simulink model "exp_dcMotor_simulink"  (R2016a)
settings: Solver=VariableStepAuto  SolverMode=SingleTasking  StartTime=0.0  StopTime=10.0  RelTol=1e-3
libraries: simulink x5
settings Model: Creator=Igor  LastModifiedBy=david
settings DebuggingCC: SFUnexpectedBacktrackingDiag=error  SFNoUnconditionalDefaultTransitionDiag=error
settings GRTTargetCC: TargetLangStandard=C99 (ISO)  GeneratePreprocessorConditionals=Use local settings
settings ConfigComp: CovMetricSettings=dwe  CovHtmlReporting=off  CovSaveCumulativeToWorkspaceVar=off  CovSaveSingleToWorkspaceVar=off  CovExternalEMLEnable=on

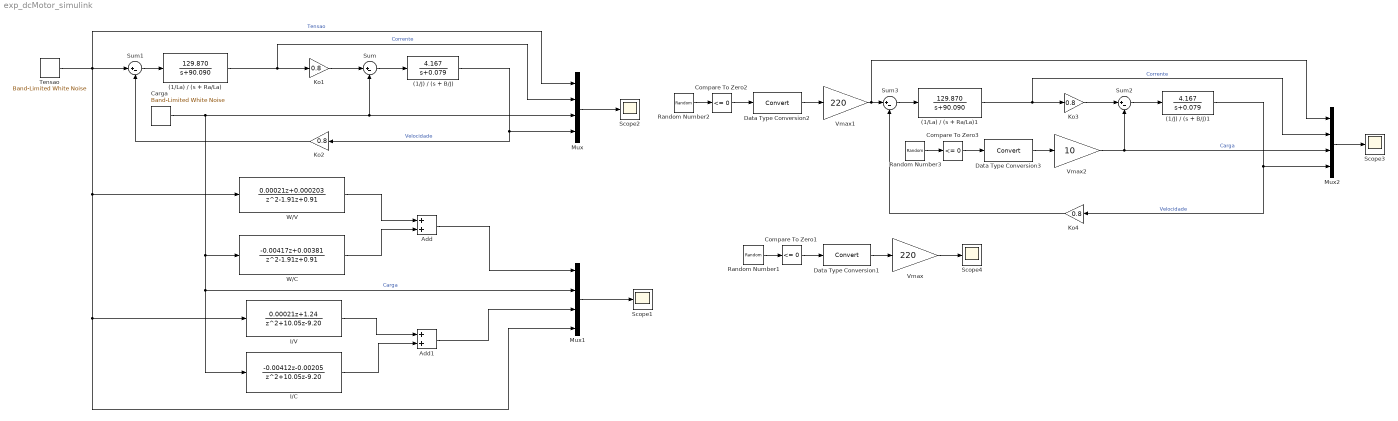
== system exp_dcMotor_simulink ==
  (1/J) / (s + B/J) : TransferFcn  Numerator=[4.167]  Denominator=[1 0.079]
  (1/J) / (s + B/J)1 : TransferFcn  Numerator=[4.167]  Denominator=[1 0.079]
  (1/La) / (s + Ra/La) : TransferFcn  Numerator=[129.870]  Denominator=[1 90.090 ]
  (1/La) / (s + Ra/La)1 : TransferFcn  Numerator=[129.870]  Denominator=[1 90.090 ]
  Add : Sum
  Add1 : Sum
  Carga : simulink/Sources/Band-Limited White Noise  Cov=[10]  Ts=0.001  seed=[23341]
  Compare To Zero1 : simulink/Logic and Bit Operations/Compare To Zero  relop=<=  OutDataTypeStr=uint8
  Compare To Zero2 : simulink/Logic and Bit Operations/Compare To Zero  relop=<=  OutDataTypeStr=uint8
  Compare To Zero3 : simulink/Logic and Bit Operations/Compare To Zero  relop=<=  OutDataTypeStr=uint8
  Data Type Conversion1 : DataTypeConversion
  Data Type Conversion2 : DataTypeConversion
  Data Type Conversion3 : DataTypeConversion
  I/C : DiscreteTransferFcn  Numerator=[-0.00412 -0.00205]  Denominator=[1 10.05 -9.20]
  "I/V " : DiscreteTransferFcn  Numerator=[0.00021 1.24]  Denominator=[1 10.05 -9.20]
  Ko{1..4} (4 alike) : Gain  Gain=0.8
  Mux : Mux
  Mux1 : Mux
  Mux2 : Mux
  Random Number1 : RandomNumber  SampleTime=0.001
  Random Number2 : RandomNumber  SampleTime=0.001
  Random Number3 : RandomNumber  SampleTime=0.001
  Scope{1..4} (4 alike) : Scope
  Sum{,1..3} (4 alike) : Sum  Inputs=|+-
  Tensao : simulink/Sources/Band-Limited White Noise  Cov=[100]  Ts=0.001  seed=[23342]
  Vmax : Gain  Gain=220
  Vmax1 : Gain  Gain=220
  Vmax2 : Gain  Gain=10
  "W/C " : DiscreteTransferFcn  Numerator=[-0.00417 0.00381]  Denominator=[1 -1.91 0.91]
  "W/V " : DiscreteTransferFcn  Numerator=[0.00021 0.000203]  Denominator=[1 -1.91 0.91]
  wires:
  Sum1/1 -> (1/La) / (s + Ra/La)/1
  (1/J) / (s + B/J)/1 -> Ko2/1, Mux/4  "Velocidade"
  Ko1/1 -> Sum/1
  Sum/1 -> (1/J) / (s + B/J)/1
  Ko2/1 -> Sum1/2
  Mux/1 -> Scope2/1
  "W/V "/1 -> Add/1
  "W/C "/1 -> Add/2
  Add/1 -> Mux1/1
  I/C/1 -> Add1/2
  "I/V "/1 -> Add1/1
  Mux1/1 -> Scope1/1
  Add1/1 -> Mux1/3
  Carga/1 -> I/C/1, Mux1/2, "W/C "/1, Sum/2, Mux/3  "Carga"
  Tensao/1 -> Mux/1, Sum1/1, "W/V "/1, Mux1/4, "I/V "/1  "Tensao"
  (1/La) / (s + Ra/La)/1 -> Ko1/1, Mux/2  "Corrente"
  Sum3/1 -> (1/La) / (s + Ra/La)1/1
  (1/J) / (s + B/J)1/1 -> Ko4/1, Mux2/4  "Velocidade"
  Ko3/1 -> Sum2/1
  Sum2/1 -> (1/J) / (s + B/J)1/1
  Ko4/1 -> Sum3/2
  Mux2/1 -> Scope3/1
  Vmax2/1 -> Sum2/2, Mux2/3  "Carga"
  (1/La) / (s + Ra/La)1/1 -> Ko3/1, Mux2/2  "Corrente"
  Random Number1/1 -> Compare To Zero1/1
  Vmax/1 -> Scope4/1
  Compare To Zero1/1 -> Data Type Conversion1/1
  Data Type Conversion1/1 -> Vmax/1
  Random Number2/1 -> Compare To Zero2/1
  Compare To Zero2/1 -> Data Type Conversion2/1
  Data Type Conversion2/1 -> Vmax1/1
  Random Number3/1 -> Compare To Zero3/1
  Compare To Zero3/1 -> Data Type Conversion3/1
  Data Type Conversion3/1 -> Vmax2/1
  Vmax1/1 -> Mux2/1, Sum3/1
